simulink model "traffic_light"  (R2023b)
settings: Solver=FixedStepDiscrete  StartTime=0.0  StopTime=inf  FixedStep=1  RelTol=1e-3
settings Model: Creator=Beshary  LastModifiedBy=Beshary

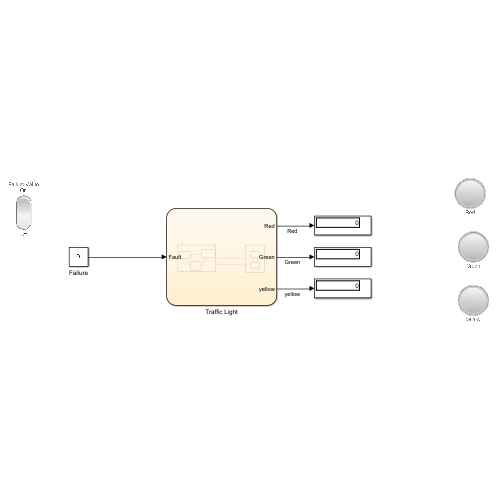
[thumbnail: Simulink's stored preview of the top-level diagram]
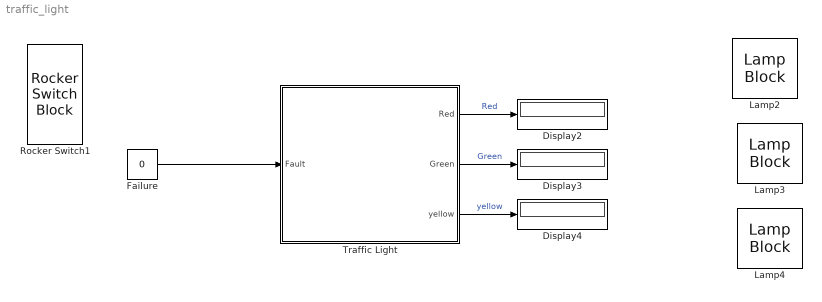
== system traffic_light ==
  Display2 : Display
  Display3 : Display
  Display4 : Display
  Failure : Constant  Value=0
  Lamp2 : LampBlock  LabelPosition=Bottom
  Lamp3 : LampBlock  LabelPosition=Bottom
  Lamp4 : LampBlock  LabelPosition=Bottom
  Rocker Switch1 : RockerSwitchBlock
      settings: Values={{'Off', 'On'}, [0 1]}
  Traffic Light : Stateflow chart  TreatAsAtomicUnit=on
  wires:
  Traffic Light/2(Green) -> Display3/1  "Green"
  Traffic Light/1(Red) -> Display2/1  "Red"
  Failure/1 -> Traffic Light/1(Fault)
  Traffic Light/3(yellow) -> Display4/1  "yellow"

== stateflow chart traffic_light/Traffic Light ==
  state Normal
    state Preparestop
      en:
      Green=0;
      Red=0;
      yellow=1;
    state Stop
      en:
      Green=0;
      Red=1;
      yellow=0;
    state GO
      en:
      Green=1;
      Red=0;
      yellow=0;
    (default) -> Stop
    Preparestop -> Stop : after(3,sec)
    GO -> Preparestop : after(4,sec)
    Stop -> GO : after(10,sec)
  state Fault
    state LedOn
      en:
      Red=1;
      yellow=0;
    state LedOff
      en:
      Red=0;
    (default) -> LedOn
    LedOn -> LedOff : after(1,sec)
    LedOff -> LedOn : after(1,sec)
  (default) -> Normal
  Normal -> Fault : [Fault==1]{Green=0}
  Fault -> Normal : [Fault==0]
  data: Fault input; Red output; Green output; yellow output
